simulink model "pc_test1"  (R2024b)
settings: Solver=FixedStepDiscrete  StartTime=0.0  StopTime=Inf  FixedStep=Ts  RelTol=1e-3  EnableMultiTasking=on
model workspace (MATLAB code in the model file):
  | % sampling time
  | 
  | fs=10000;
  | Ts=1/fs;
libraries: instrumentseriallib x3, svdutilitieslib x1, instrumentlib x1
settings Model: ExtModeTrigDuration=8  Creator=The MathWorks, Inc.  LastModifiedBy=nicvi
settings SolverCC: AlgebraicLoopSolver=TrustRegion
settings OptimizationCC: DefaultUnderspecifiedDataType=single  EnhancedBackFolding=on  PassReuseOutputArgsAs=Individual arguments  MaxStackSize=1024  OptimizeBlockOrder=speed  DifferentSizesBufferReuse=on  OptimizationCustomize=off  DenormalBehavior=FlushToZero  EfficientTunableParamExpr=on
settings DebuggingCC: ParameterTunabilityLossMsg=error  UnconnectedInputMsg=warning  UnconnectedOutputMsg=warning  UnconnectedLineMsg=warning  SubsystemReferenceDiagnosticForUnitTest=warning
settings HardwareCC: ProdBitPerChar=16  ProdBitPerInt=16  ProdBitPerPointer=32  ProdBitPerSizeT=32  ProdBitPerPtrDiffT=32  ProdLargestAtomicInteger=Integer  ProdLargestAtomicFloat=None  ProdWordSize=16  ProdLongLongMode=on  ProdHWDeviceType=Texas Instruments->C2000
settings ModelReferenceCC: EnableRefExpFcnMdlSchedulingChecks=on
settings SFSimCC: MATLABDynamicMemAlloc=off
settings RTWCC: Description=Embedded Coder  SystemTargetFile=ert.tlc  HardwareBoard=TI Piccolo F28069M LaunchPad  TemplateMakefile=ert_default_tmf  GenerateReport=on  Toolchain=Texas Instruments Code Composer Studio (C2000)  GPUComputeCapability=3.5  DLArmComputeVersion=19.05
settings CodeAppCC: ForceParamTrailComments=on  IgnoreCustomStorageClasses=off  OperatorAnnotations=on  SimulinkDataObjDesc=on  SFDataObjDesc=on  InsertBlockDesc=on
settings ERTTargetCC: CodeReplacementLibrary=TI C28x  ExtModeStaticAllocSize=2000  InlinedParameterPlacement=Hierarchical  DynamicArrayContainerType=coder::array

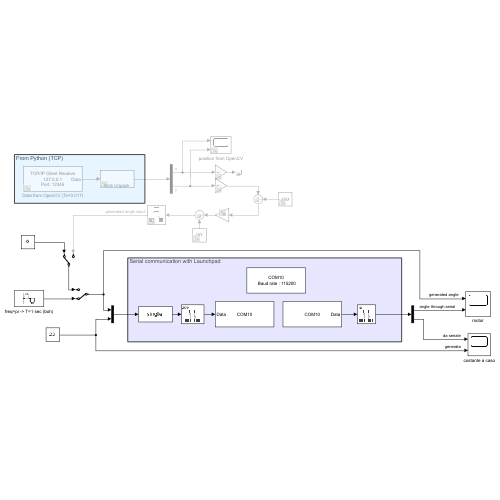
[thumbnail: Simulink's stored preview of the top-level diagram]
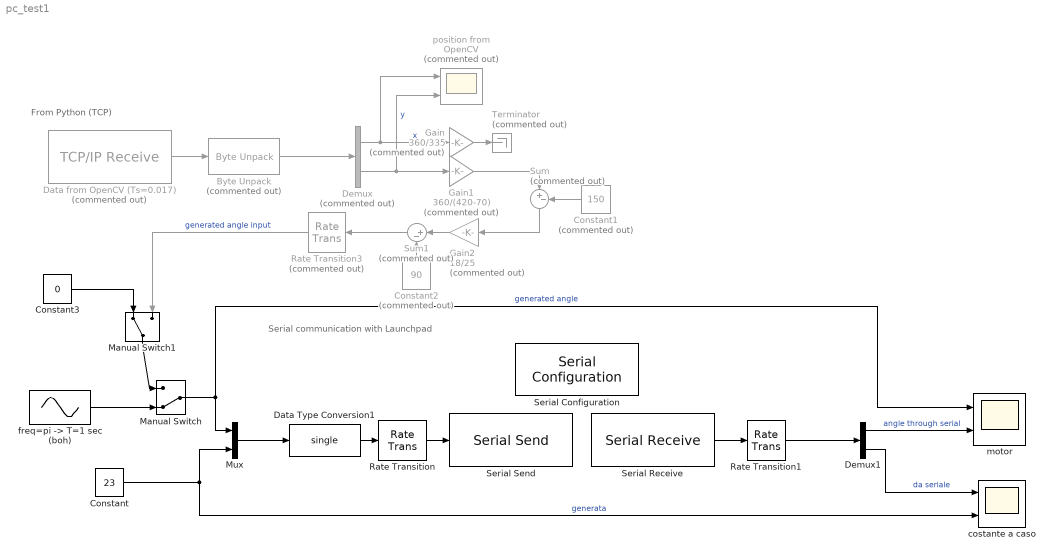
== system pc_test1 ==
  note: From Python (TCP)
  note: Serial communication with Launchpad
  Byte Unpack : svdutilitieslib/Byte Unpack  Commented=on  dimensions={[2]}  datatypes={'uint16'}  byteAlign=4  blockPlatform=tic2000
      settings: LibrarySourceBlock=c2000lib/Target Communication/Byte Unpack
  Constant : Constant  Value=23
  Constant1 : Constant  Commented=on  Value=150
  Constant2 : Constant  Commented=on  Value=90
  Constant3 : Constant  Value=0
  Data Type Conversion1 : DataTypeConversion  OutDataTypeStr=single  SaturateOnIntegerOverflow=off  RndMeth=Floor
  Data from OpenCV (Ts=0.017) : instrumentlib/TCP//IP Receive  Commented=on  Host=127.0.0.1  Port=12345  DataSize=2  DataType=uint16  ASCIIFormatting=%f  Terminator=LF  CustomTerminator=10  ByteOrder=big-endian  EnableBlockingMode=on  Timeout=10  SampleTime=0.0167*2  SimulateUsing=Interpreted execution
  Demux : Demux  Commented=on  Outputs=2
  Demux1 : Demux  Outputs=2
  Gain : Gain  Commented=on  Gain=360/335
  Gain1 : Gain  Commented=on  Gain=360/(420-70)
  Gain2 : Gain  Commented=on  Gain=18/25
  Manual Switch : ManualSwitch  CurrentSetting=0
  Manual Switch1 : ManualSwitch
  Mux : Mux  Inputs=2
  Rate Transition : RateTransition  OutPortSampleTime=100*Ts
  Rate Transition1 : RateTransition  OutPortSampleTime=Ts
  Rate Transition3 : RateTransition  Commented=on  OutPortSampleTime=Ts
  Serial Configuration : instrumentseriallib/Serial Configuration  Priority=-200000  PortSel=COM10  Port=COM10  ComPort=COM10  BaudRate=115200  DataBits=8  Parity=none  StopBits=1  ByteOrder=little-endian  FlowControl=none  Timeout=10  SimulateUsing=Interpreted execution  BlockInModel=on  aMode=1
      settings: LibrarySourceBlock=c2000lib/Host Communication/Serial Configuration
  Serial Receive : instrumentseriallib/Serial Receive  Priority=1  PortSel=COM10  Port=COM10  ComPort=COM10  DataType=single  SaveDataType=uint8  ToggleHeader=off  Header=[]  ToggleDataSize=on  DataSize=2  ToggleTerminator=off  Terminator=<none>  CustomTerminator=[]  InputFormat=Column major  EnableBlockingMode=on  ActionDataUnavailable=Output last received value  ActionWhenDataUnavailable=Output last received value  CustomValue=100  SampleTime=100*Ts  SimulateUsing=Interpreted execution  BlockInModel=on  aMode=1
      settings: LibrarySourceBlock=c2000lib/Host Communication/Serial Receive
  Serial Send : instrumentseriallib/Serial Send  Priority=1  PortSel=COM10  Port=COM10  ComPort=COM10  Header=[]  Terminator=<none>  CustomTerminator=[]  EnableBlockingMode=on  SimulateUsing=Interpreted execution  BlockInModel=on  aMode=1
      settings: LibrarySourceBlock=c2000lib/Host Communication/Serial Send
  Sum : Sum  Commented=on  Inputs=|+-
  Sum1 : Sum  Commented=on  Inputs=|+-
  Terminator : Terminator  Commented=on
  costante a caso : Scope  NumInputPorts=2
  "freq=pi -> T=1 sec (boh)" : Sin  Amplitude=45  Frequency=2*pi  SampleTime=1/fs
  motor : Scope  NumInputPorts=2
  position from OpenCV : Scope  Commented=on  NumInputPorts=2
  wires:
  Serial Receive/1 -> Rate Transition1/1
  Rate Transition/1 -> Serial Send/1
  Data Type Conversion1/1 -> Rate Transition/1
  Demux/1 -> Gain/1, position from OpenCV/1  "x"
  Demux/2 -> Gain1/1, position from OpenCV/2  "y"
  Rate Transition3/1 -> Manual Switch1/2  "generated angle input"
  Mux/1 -> Data Type Conversion1/1
  Gain/1 -> Terminator/1
  Constant/1 -> costante a caso/2, Mux/2  "generata"
  Rate Transition1/1 -> Demux1/1
  Demux1/1 -> motor/2  "angle through serial"
  Demux1/2 -> costante a caso/1  "da seriale"
  "freq=pi -> T=1 sec (boh)"/1 -> Manual Switch/2
  Constant1/1 -> Sum/2
  Gain1/1 -> Sum/1
  Sum/1 -> Gain2/1
  Gain2/1 -> Sum1/1
  Constant2/1 -> Sum1/2
  Manual Switch/1 -> Mux/1, motor/1  "generated angle"
  Sum1/1 -> Rate Transition3/1
  Constant3/1 -> Manual Switch1/1
  Manual Switch1/1 -> Manual Switch/1
  Byte Unpack/1 -> Demux/1
  Data from OpenCV (Ts=0.017)/1 -> Byte Unpack/1
